simulink model "TryingToAnimate1"  (R2023b)
settings: Solver=VariableStepAuto  StartTime=0.0  StopTime=10  RelTol=1e-3
values from neighbouring files (symbols this model uses):
  A = [0 1 0 0; 0 a1 a2 0;0 0 0 1;0 a3 a4 0]    [TryingToAnimate.m]
  B = [0; ((I+m*l^2)*Kt*r)/(d*Rm); 0; (-m*l*r*Kt)/(d*Rm)]    [TryingToAnimate.m]
  Ts = 0.03    [TryingToAnimate.m]
  x0 = [0; 0; 0.05; 0.1]    [TryingToAnimate.m]
undefined symbols (not defined in the file or in its folder): K_d
settings Model: Creator=biswa  LastModifiedBy=biswa

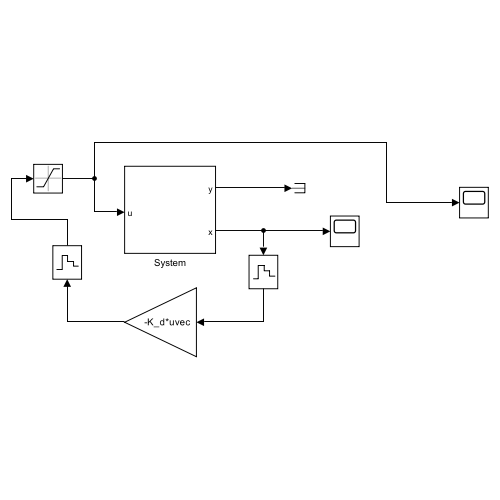
[thumbnail: Simulink's stored preview of the top-level diagram]
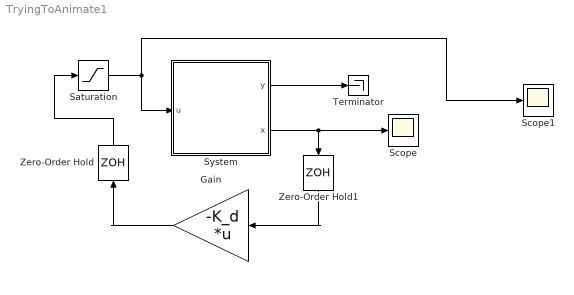
== system TryingToAnimate1 ==
  Gain : Gain  Gain=-K_d  Multiplication=Matrix(K*u) (u vector)
  Saturation : Saturate  UpperLimit=12  LowerLimit=-12
  Scope : Scope
  Scope1 : Scope
  System : Subsystem
  Terminator : Terminator
  Zero-Order Hold : ZeroOrderHold  SampleTime=Ts
  Zero-Order Hold1 : ZeroOrderHold  SampleTime=Ts
  wires:
  Gain/1 -> Zero-Order Hold/1
  System/1(y) -> Terminator/1
  System/2(x) -> Scope/1, Zero-Order Hold1/1
  Zero-Order Hold1/1 -> Gain/1
  Zero-Order Hold/1 -> Saturation/1
  Saturation/1 -> Scope1/1, System/1(u)

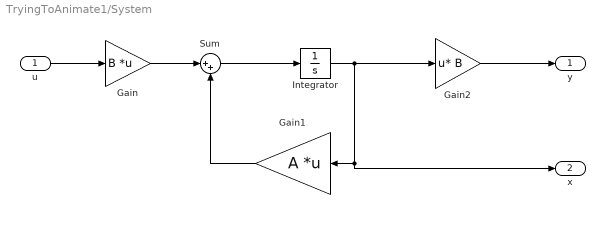
== system TryingToAnimate1/System ==
  u : Inport
  Gain : Gain  Gain=B  Multiplication=Matrix(K*u)
  Gain1 : Gain  Gain=A  Multiplication=Matrix(K*u) (u vector)
  Gain2 : Gain  Gain=B  Multiplication=Matrix(u*K)
  Integrator : Integrator  InitialCondition=x0
  Sum : Sum  Inputs=|++
  y : Outport
  x : Outport  Port=2
  wires:
  Sum/1 -> Integrator/1
  Integrator/1 -> Gain2/1, x/1, Gain1/1
  Gain/1 -> Sum/1
  Gain1/1 -> Sum/2
  Gain2/1 -> y/1
  u/1 -> Gain/1
